simulink subsystem "SimscapePlantModels"  (R2023b)
settings: Solver=VariableStepAuto  StartTime=0.0  StopTime=10.0  RelTol=1e-3
undefined symbols (not defined in the file or in its folder): AxlFL, AxlFR, AxlRL, AxlRR, PlntTrnsfrCaseAxlSpdLock, PlntTrnsfrCaseTrqSplitRatio
libraries: fl_lib x13, nesl_utility_internal x9, sdl_lib x3, simulink x2, nesl_utility x2
(part 1 of 2)
settings Model: ModifiedByFormat=The MathWorks, Inc.  Creator=The MathWorks, Inc.  LastModifiedBy=The MathWorks, Inc.
settings SolverCC: MaxZcPerStep=1
settings OptimizationCC: ReuseModelBlockBuffer=off
settings DebuggingCC: UnconnectedInputMsg=warning  UnconnectedOutputMsg=warning  UnconnectedLineMsg=warning  SubsystemReferenceDiagnosticForUnitTest=warning
settings ModelReferenceCC: EnableRefExpFcnMdlSchedulingChecks=on
settings RTWCC: DLArmComputeVersion=19.05

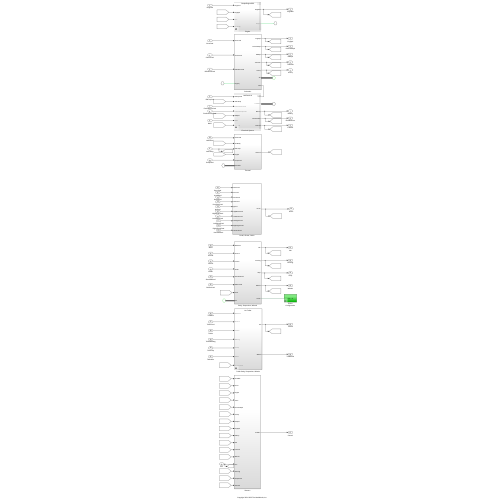
[thumbnail: Simulink's stored preview of the top-level diagram]
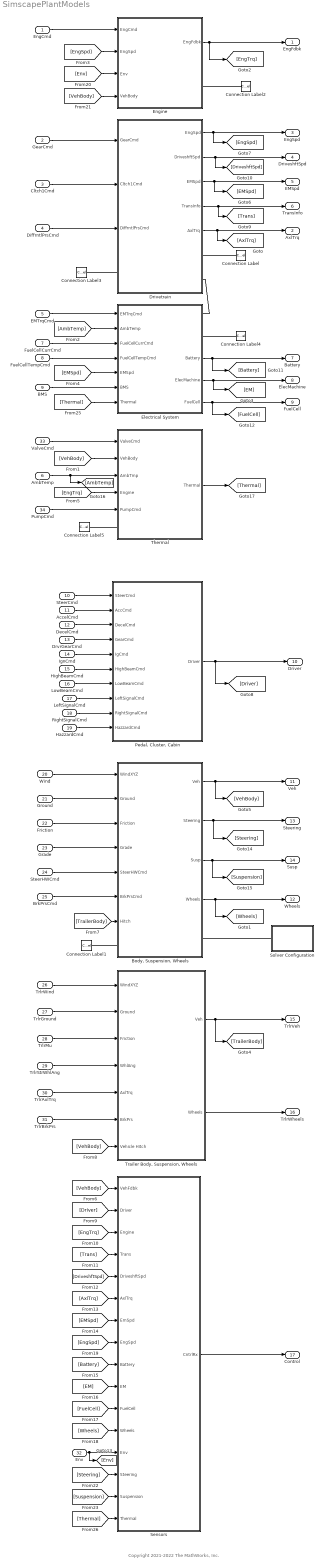
== system SimscapePlantModels ==
  note: Copyright 2021-2022 The MathWorks, Inc.
  EngCmd : Inport
  GearCmd : Inport  Port=2
  Cltch1Cmd : Inport  Port=3
  DiffrntlPrsCmd : Inport  Port=4
  EMTrqCmd : Inport  Port=5
  AmbTemp : Inport  Port=6
  FuelCellCurrCmd : Inport  Port=7
  FuelCellTempCmd : Inport  Port=8
  BMS : Inport  Port=9
  SteerCmd : Inport  Port=10
  AccelCmd : Inport  Port=11
  DecelCmd : Inport  Port=12
  DrvrGearCmd : Inport  Port=13
  IgnCmd : Inport  Port=14
  HighBeamCmd : Inport  Port=15
  LowBeamCmd : Inport  Port=16
  LeftSignalCmd : Inport  Port=17
  RightSignalCmd : Inport  Port=18
  HazzardCmd : Inport  Port=19
  Wind : Inport  Port=20
  Ground : Inport  Port=21
  Friction : Inport  Port=22
  Grade : Inport  Port=23
  SteerHWCmd : Inport  Port=24
  BrkPrsCmd : Inport  Port=25
  TrlrWind : Inport  Port=26
  TrlrGround : Inport  Port=27
  TrlrMu : Inport  Port=28
  TrlrStrWhlAng : Inport  Port=29
  TrlrAxlTrq : Inport  Port=30
  TrlrBrkPrs : Inport  Port=31
  Env : Inport  Port=32
  ValveCmd : Inport  Port=33
  PumpCmd : Inport  Port=34
  "Body, Suspension, Wheels" : Subsystem  VariantControl=Longitudinal Vehicle Dynamics
  Connection Label : ConnectionLabel  Label=Axl
  Connection Label1 : ConnectionLabel  Label=Axl
  Connection Label2 : ConnectionLabel  Label=EngTrq
  Connection Label3 : ConnectionLabel  Label=EngTrq
  Connection Label4 : ConnectionLabel  Label=ThrmElec
  Connection Label5 : ConnectionLabel  Label=ThrmElec
  Drivetrain : Subsystem
  Electrical System : Subsystem  Variant=on  VariantChoicesSpecifier={'ElectricalSystemSSC', 'NoElectrical'}  VariantControlMode=label  VariantControl=Choice  LabelModeActiveChoice=NoElectrical
      settings: PortSchema="{\"entries\":[{\"content\":{\"sides\":[{\"content\":{\"connectorIds\":[\"In1\",\"In2\",\"In3\",\"In4\",\"In5\",\"In6\",\"In7\"]},\"type\":\"ConnectorPlacement.EquallySpacedRectSide\",\"uuid\":\"168fda7d-02fd-4045-80e4-d70d0b749a9c\"},{\"content\":{\"connectorIds\":[\"RConn1\",\"RConn2\",\"Out1\",\"Out2\",\"Out3\"],\"side\":\"RIGHT\"},\"type\":\"ConnectorPlacement.EquallySpacedRectSide\",\"uuid\":\"a7e9bf4a-b9ce-46d6-8afc-0075c6e03a0c\"},{\"content\":{\"side\":\"TOP\"},\"type\":\"ConnectorPlacement.EquallySpacedRectSide\",\"uuid\":\"81c60468-d7ed-4851-a727-3a9a5b008640\"}]},\"type\":\"ConnectorPlacement.EquallySpacedConnector\",\"uuid\":\"8c7c8f28-264e-479c-b2d0-01b49dca4966\"}],\"packageUris\":[\"http://schema.mathworks.com/mf0/Connector/R2020b\"],\"version\":\"1.0\"}"
  Engine : Subsystem  Variant=on  VariantChoicesSpecifier={'FMUEngineSSC', 'NoEngine', 'SimpleEngineSSC'}  VariantControlMode=label  LabelModeActiveChoice=SimpleEngineSSC
  "Pedal, Cluster, Cabin" : Subsystem
  Sensors : Subsystem
  Solver Configuration : Subsystem  Variant=on  VariantControlMode=label  VariantControl=Choice  LabelModeActiveChoice=Solver Configuration
  Thermal : Subsystem
  "Trailer Body, Suspension, Wheels" : Subsystem  Variant=on  VariantControlMode=label  LabelModeActiveChoice=No Trailer
  EngFdbk : Outport
  AxlTrq : Outport  Port=2
  EngSpd : Outport  Port=3
  DriveshftSpd : Outport  Port=4
  EMSpd : Outport  Port=5
  TransInfo : Outport  Port=6
  Battery : Outport  Port=7
  ElecMachine : Outport  Port=8
  FuelCell : Outport  Port=9
  Driver : Outport  Port=10
  Veh : Outport  Port=11
  Wheels : Outport  Port=12
  Steering : Outport  Port=13
  Susp : Outport  Port=14
  TrlrVeh : Outport  Port=15
  TrlrWheels : Outport  Port=16
  Control : Outport  Port=17
  wires:
  Drivetrain/4(TransInfo) -> [Trans], TransInfo/1
  EngCmd/1 -> Engine/1(EngCmd)
  Electrical System/3(FuelCell) -> FuelCell/1, [FuelCell]
  Electrical System/1(Battery) -> Battery/1, [Battery]
  TrlrGround/1 -> "Trailer Body, Suspension, Wheels"/2(Ground)
  Wind/1 -> "Body, Suspension, Wheels"/1(WindXYZ)
  TrlrAxlTrq/1 -> "Trailer Body, Suspension, Wheels"/5(AxlTrq)
  EMTrqCmd/1 -> Electrical System/1(EMTrqCmd)
  DiffrntlPrsCmd/1 -> Drivetrain/3(DiffrntlPrsCmd)
  TrlrMu/1 -> "Trailer Body, Suspension, Wheels"/3(Friction)
  Friction/1 -> "Body, Suspension, Wheels"/3(Friction)
  SteerHWCmd/1 -> "Body, Suspension, Wheels"/5(SteerHWCmd)
  [EMSpd] -> Electrical System/5(EMSpd)
  Ground/1 -> "Body, Suspension, Wheels"/2(Ground)
  SteerCmd/1 -> "Pedal, Cluster, Cabin"/1(SteerCmd)
  TrlrBrkPrs/1 -> "Trailer Body, Suspension, Wheels"/6(BrkPrs)
  Drivetrain/2(DriveshftSpd) -> [DriveshftSpd], DriveshftSpd/1
  "Body, Suspension, Wheels"/1(Veh) -> [VehBody], Veh/1
  Engine/1(EngFdbk) -> [EngTrq], EngFdbk/1
  BrkPrsCmd/1 -> "Body, Suspension, Wheels"/6(BrkPrsCmd)
  Cltch1Cmd/1 -> Drivetrain/2(Cltch1Cmd)
  TrlrWind/1 -> "Trailer Body, Suspension, Wheels"/1(WindXYZ)
  TrlrStrWhlAng/1 -> "Trailer Body, Suspension, Wheels"/4(WhlAng)
  [VehBody] -> "Trailer Body, Suspension, Wheels"/7(Vehicle Hitch)
  "Trailer Body, Suspension, Wheels"/2(Wheels) -> TrlrWheels/1
  Electrical System/2(ElecMachine) -> ElecMachine/1, [EM]
  [TrailerBody] -> "Body, Suspension, Wheels"/7(Hitch)
  DecelCmd/1 -> "Pedal, Cluster, Cabin"/3(DecelCmd)
  DrvrGearCmd/1 -> "Pedal, Cluster, Cabin"/4(GearCmd)
  Drivetrain/3(EMSpd) -> [EMSpd], EMSpd/1
  IgnCmd/1 -> "Pedal, Cluster, Cabin"/5(IgCmd)
  FuelCellTempCmd/1 -> Electrical System/4(FuelCellTempCmd)
  GearCmd/1 -> Drivetrain/1(GearCmd)
  "Body, Suspension, Wheels"/4(Wheels) -> [Wheels], Wheels/1
  "Trailer Body, Suspension, Wheels"/1(Veh) -> TrlrVeh/1, [TrailerBody]
  FuelCellCurrCmd/1 -> Electrical System/3(FuelCellCurrCmd)
  AccelCmd/1 -> "Pedal, Cluster, Cabin"/2(AccCmd)
  Drivetrain/1(EngSpd) -> EngSpd/1, [EngSpd]
  [VehBody] -> Sensors/1(VehFdbk)
  "Pedal, Cluster, Cabin"/1(Driver) -> Driver/1, [Driver]
  [Driver] -> Sensors/2(Driver)
  [EngTrq] -> Sensors/3(Engine)
  [Trans] -> Sensors/4(Trans)
  [DriveshftSpd] -> Sensors/5(DriveshftSpd)
  [AxlTrq] -> Sensors/6(AxlTrq)
  [EMSpd] -> Sensors/7(EmSpd)
  [Battery] -> Sensors/9(Battery)
  [EM] -> Sensors/10(EM)
  [FuelCell] -> Sensors/11(FuelCell)
  [Wheels] -> Sensors/12(Wheels)
  Sensors/1(CntrlRx) -> Control/1
  Env/1 -> [Env], Sensors/13(Env)
  [EngSpd] -> Sensors/8(EngSpd)
  [Env] -> Engine/3(Env)
  [VehBody] -> Engine/4(VehBody)
  [EngSpd] -> Engine/2(EngSpd)
  "Body, Suspension, Wheels"/3(Susp) -> [Suspension], Susp/1
  Grade/1 -> "Body, Suspension, Wheels"/4(Grade)
  Drivetrain/5(AxlTrq) -> [AxlTrq], AxlTrq/1
  BMS/1 -> Electrical System/6(BMS)
  [Steering] -> Sensors/14(Steering)
  [Suspension] -> Sensors/15(Suspension)
  "Body, Suspension, Wheels"/2(Steering) -> [Steering], Steering/1
  Thermal/1(Thermal) -> [Thermal]
  [VehBody] -> Thermal/2(VehBody)
  ValveCmd/1 -> Thermal/1(ValveCmd)
  [EngTrq] -> Thermal/4(Engine)
  AmbTemp/1 -> [AmbTemp], Thermal/3(AmbTmp)
  [AmbTemp] -> Electrical System/2(AmbTemp)
  [Thermal] -> Electrical System/7(Thermal)
  [Thermal] -> Sensors/16(Thermal)
  PumpCmd/1 -> Thermal/5(PumpCmd)
  RightSignalCmd/1 -> "Pedal, Cluster, Cabin"/9(RightSignalCmd)
  LowBeamCmd/1 -> "Pedal, Cluster, Cabin"/7(LowBeamCmd)
  HighBeamCmd/1 -> "Pedal, Cluster, Cabin"/6(HighBeamCmd)
  HazzardCmd/1 -> "Pedal, Cluster, Cabin"/10(HazzardCmd)
  LeftSignalCmd/1 -> "Pedal, Cluster, Cabin"/8(LeftSignalCmd)
  connections:
  Connection Label/LConn1 -- Drivetrain/RConn1
  "Body, Suspension, Wheels"/LConn1 -- Connection Label1/LConn1
  Electrical System/RConn1 -- Drivetrain/RConn2
  Drivetrain/LConn1 -- Connection Label3/LConn1
  Connection Label2/LConn1 -- Engine/RConn1
  Solver Configuration/RConn1 -- "Body, Suspension, Wheels"/RConn1
  Thermal/LConn1 -- Connection Label5/LConn1
  Connection Label4/LConn1 -- Electrical System/RConn2

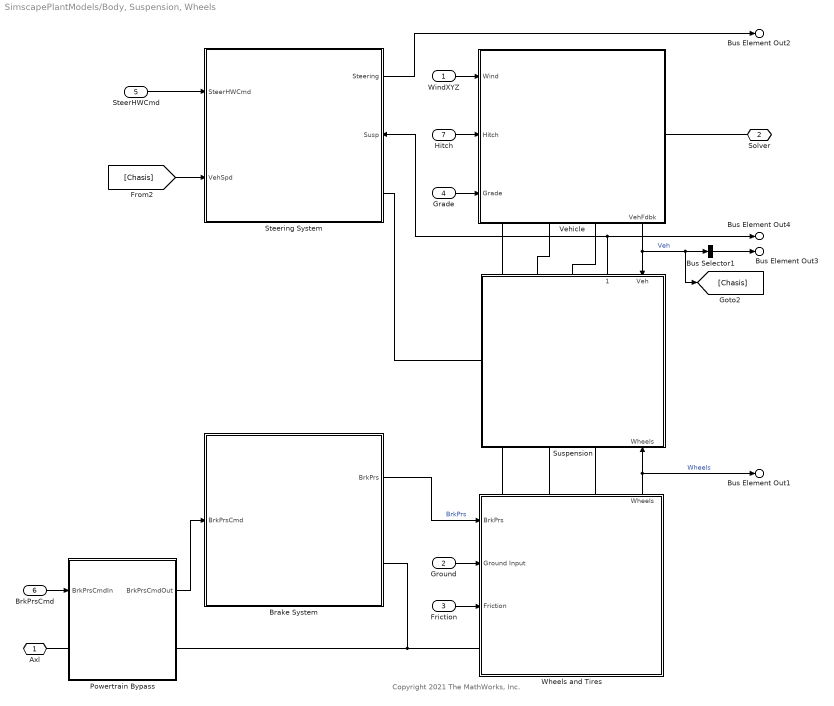
== system SimscapePlantModels/Body, Suspension, Wheels ==
  note: Copyright 2021 The MathWorks, Inc.
  WindXYZ : Inport  Unit=m/s  PortDimensions=3
  Ground : Inport  Port=2  Unit=m  PortDimensions=4
  Friction : Inport  Port=3  Unit=1  PortDimensions=4
  Grade : Inport  Port=4  Unit=deg  PortDimensions=1
  SteerHWCmd : Inport  Port=5  Unit=rad
  BrkPrsCmd : Inport  Port=6  PortDimensions=4
  Hitch : Inport  Port=7
  Brake System : Subsystem  Variant=on  VariantControlMode=label  VariantControl=Choice  LabelModeActiveChoice=Braking Hydraulics and Disc Brakes
      mask Display: image('Caliper.png',[.125,.125,.75,.75])
  Bus Selector1 : BusSelector  OutputSignals=InertFrm,BdyFrm  OutputAsBus=on
  Powertrain Bypass : Subsystem  Variant=on  VariantControlMode=label  VariantControl=Choice  LabelModeActiveChoice=Pass Through
  Steering System : Subsystem  Variant=on  VariantChoicesSpecifier={'NoSteering', 'SteeringSystemSSC'}  VariantControlMode=label  VariantControl=0  LabelModeActiveChoice=NoSteering
      settings: PortSchema="{\"entries\":[{\"content\":{\"sides\":[{\"content\":{\"connectorIds\":[\"In1\",\"In2\"]},\"type\":\"ConnectorPlacement.EquallySpacedRectSide\",\"uuid\":\"f4eae9a1-ee72-4894-9c3f-d81ee40fba89\"},{\"content\":{\"connectorIds\":[\"Out1\",\"In3\",\"RConn1\"],\"side\":\"RIGHT\"},\"type\":\"ConnectorPlacement.EquallySpacedRectSide\",\"uuid\":\"c62a78d9-dc5d-4f96-a554-c82d7fa22a9e\"},{\"content\":{\"side\":\"TOP\"},\"type\":\"ConnectorPlacement.EquallySpacedRectSide\",\"uuid\":\"38f3851a-1d1e-4a2b-8c09-8e5c8dcc7723\"}]},\"type\":\"ConnectorPlacement.EquallySpacedConnector\",\"uuid\":\"9f269846-92fa-4948-bc2b-71154f41fdde\"}],\"packageUris\":[\"http://schema.mathworks.com/mf0/Connector/R2020b\"],\"version\":\"1.0\"}"
      mask Display:
      | switch get_param(gcb,'ActiveVariant')
      |     case 'Kinematic Steering'
      |         image('KinematicSteering.png');
      |     case 'Mapped Steering'
      |         image('MappedSteering.png');
      |     case 'Dynamic Steering'
      |         image('DynamicSteering.png');
      |     otherwise
      |         image('DynamicSteering.png');
      | end
  Suspension : Subsystem  Variant=on  VariantChoicesSpecifier={'MultibodySuspensionSSC', 'NoSuspensionSSC'}  VariantControlMode=label  VariantControl=Choice  LabelModeActiveChoice=NoSuspensionSSC
      settings: PortSchema="{\"entries\":[{\"content\":{\"sides\":[{\"content\":{\"connectorIds\":[\"LConn1\"]},\"type\":\"ConnectorPlacement.EquallySpacedRectSide\",\"uuid\":\"0a9265e3-f55e-4b74-9b74-681dc9522591\"},{\"content\":{\"side\":\"RIGHT\"},\"type\":\"ConnectorPlacement.EquallySpacedRectSide\",\"uuid\":\"92df639a-7bc2-4e90-97ea-0cb216e2f16a\"},{\"content\":{\"connectorIds\":[\"LConn2\",\"LConn3\",\"LConn4\",\"Out1\",\"In1\"],\"side\":\"TOP\"},\"type\":\"ConnectorPlacement.EquallySpacedRectSide\",\"uuid\":\"2064b6cb-c7a8-4cfb-82de-a07750d990cb\"},{\"content\":{\"connectorIds\":[\"RConn1\",\"RConn2\",\"RConn3\",\"In2\"],\"side\":\"BOTTOM\"},\"type\":\"ConnectorPlacement.EquallySpacedRectSide\",\"uuid\":\"169bd4e6-c3fe-4e36-acea-c25875014463\"}]},\"type\":\"ConnectorPlacement.EquallySpacedConnector\",\"uuid\":\"e0b50182-0637-4594-80e7-4ddd0df85797\"}],\"packageUris\":[\"http://schema.mathworks.com/mf0/Connector/R2020b\"],\"version\":\"1.0\"}"
      mask Display:
      | switch get_param(gcb,'ActiveVariant')
      |     case 'Kinematics and Compliance Independent Suspension'
      |         image('KandCSuspension.png');
      |     case 'Kinematics and Compliance Twist Beam Suspension'
      |         image('KandCSuspensionTwistBeam.png');
      |     case 'MacPherson Front Suspension Solid Axle Rear Suspension'
      |         image([imread('suspmacp.png');imread('suspsacoil.png')]);
      |     otherwise
      |         image([imread('suspmacp.png');imread('suspsacoil.png')]);
      | end
  Vehicle : Subsystem  Variant=on  VariantChoicesSpecifier={'VehicleBody1DOFLongitudinalSSC', 'VehicleBody3DOFLongitudinalSSC', 'VehicleBody6DOFSSC'}  VariantControlMode=label  VariantControl=Choice  LabelModeActiveChoice=VehicleBody3DOFLongitudinalSSC
      settings: PortSchema="{\"entries\":[{\"content\":{\"sides\":[{\"content\":{\"connectorIds\":[\"In1\",\"In2\",\"In3\"]},\"type\":\"ConnectorPlacement.EquallySpacedRectSide\",\"uuid\":\"0a9265e3-f55e-4b74-9b74-681dc9522591\"},{\"content\":{\"connectorIds\":[\"RConn1\"],\"side\":\"RIGHT\"},\"type\":\"ConnectorPlacement.EquallySpacedRectSide\",\"uuid\":\"92df639a-7bc2-4e90-97ea-0cb216e2f16a\"},{\"content\":{\"connectorIds\":[],\"side\":\"TOP\"},\"type\":\"ConnectorPlacement.EquallySpacedRectSide\",\"uuid\":\"2064b6cb-c7a8-4cfb-82de-a07750d990cb\"},{\"content\":{\"connectorIds\":[\"RConn2\",\"RConn3\",\"RConn4\",\"Out1\"],\"side\":\"BOTTOM\"},\"type\":\"ConnectorPlacement.EquallySpacedRectSide\",\"uuid\":\"2b34afca-0a88-43db-924f-6476183b84bd\"}]},\"type\":\"ConnectorPlacement.EquallySpacedConnector\",\"uuid\":\"e0b50182-0637-4594-80e7-4ddd0df85797\"}],\"packageUris\":[\"http://schema.mathworks.com/mf0/Connector/R2020b\"],\"version\":\"1.0\"}"
      mask Display: image('6dofcar.png');
  Wheels and Tires : Subsystem  Variant=on  VariantChoicesSpecifier={'MFTiresLongitudinalSSC', 'MFTiresMultibodySSC'}  VariantControlMode=label  VariantControl=Choice  LabelModeActiveChoice=MFTiresLongitudinalSSC
      settings: PortSchema="{\"entries\":[{\"content\":{\"sides\":[{\"content\":{\"connectorIds\":[\"In1\",\"In2\",\"In3\",\"LConn1\"]},\"type\":\"ConnectorPlacement.EquallySpacedRectSide\",\"uuid\":\"fdb4d4cd-d0c0-42d9-b073-775af31e96a1\"},{\"content\":{\"connectorIds\":[],\"side\":\"RIGHT\"},\"type\":\"ConnectorPlacement.EquallySpacedRectSide\",\"uuid\":\"04106ddf-9917-4cd4-b177-ae763d642686\"},{\"content\":{\"connectorIds\":[\"LConn2\",\"LConn3\",\"LConn4\",\"Out1\"],\"side\":\"TOP\"},\"type\":\"ConnectorPlacement.EquallySpacedRectSide\",\"uuid\":\"568bf95c-0e25-4c45-a134-c198357b75be\"}]},\"type\":\"ConnectorPlacement.EquallySpacedConnector\",\"uuid\":\"4f44df5e-0d14-43ea-934e-2abe86546e95\"}],\"packageUris\":[\"http://schema.mathworks.com/mf0/Connector/R2020b\"],\"version\":\"1.0\"}"
      mask Display: image('wheel3dof.png')
  Axl : PMIOPort  Side=Left
  Solver : PMIOPort  Port=2  Side=Right
  Bus Element Out3 : Outport  PortName=Veh
  Bus Element Out2 : Outport  Port=2  PortName=Steering
  Bus Element Out4 : Outport  Port=3  PortName=Susp
  Bus Element Out1 : Outport  Port=4  PortName=Wheels
  wires:
  SteerHWCmd/1 -> Steering System/1(SteerHWCmd)
  Bus Selector1/1 -> Bus Element Out3/1
  WindXYZ/1 -> Vehicle/1(Wind)
  Brake System/1(BrkPrs) -> Wheels and Tires/1(BrkPrs)  "BrkPrs"
  Suspension/1(SuspChassis) -> Bus Element Out4/1, Steering System/3(Susp)
  Powertrain Bypass/1(BrkPrsCmdOut) -> Brake System/1(BrkPrsCmd)
  Wheels and Tires/1(Wheels) -> Bus Element Out1/1, Suspension/2(Wheels)  "Wheels"
  Grade/1 -> Vehicle/3(Grade)
  Hitch/1 -> Vehicle/2(Hitch)
  Friction/1 -> Wheels and Tires/3(Friction)
  Steering System/1(Steering) -> Bus Element Out2/1
  [Chasis] -> Steering System/2(VehSpd)
  Ground/1 -> Wheels and Tires/2(Ground Input)
  Vehicle/1(VehFdbk) -> [Chasis], Bus Selector1/1, Suspension/1(Veh)  "Veh"
  BrkPrsCmd/1 -> Powertrain Bypass/1(BrkPrsCmdIn)
  connections:
  Brake System/RConn1 -- Powertrain Bypass/RConn1 -- Wheels and Tires/LConn1
  Vehicle/RConn2 -- Suspension/LConn2
  Vehicle/RConn3 -- Suspension/LConn3
  Vehicle/RConn4 -- Suspension/LConn4
  Wheels and Tires/LConn2 -- Suspension/RConn1
  Wheels and Tires/LConn3 -- Suspension/RConn2
  Wheels and Tires/LConn4 -- Suspension/RConn3
  Vehicle/RConn1 -- Solver/RConn1
  Axl/RConn1 -- Powertrain Bypass/LConn1
  Steering System/RConn1 -- Suspension/LConn1

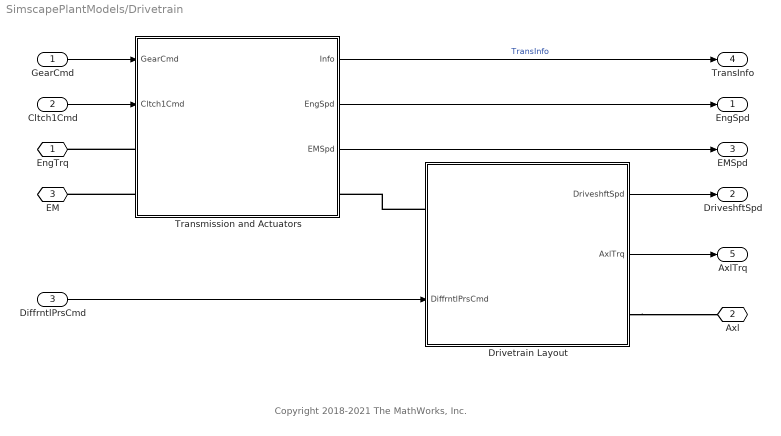
== system SimscapePlantModels/Drivetrain ==
  note: Copyright 2018-2021 The MathWorks, Inc.
  GearCmd : Inport
  Cltch1Cmd : Inport  Port=2
  DiffrntlPrsCmd : Inport  Port=3
  Drivetrain Layout : Subsystem  VariantControl=New
      settings: PortSchema="{\"entries\":[{\"content\":{\"sides\":[{\"content\":{\"connectorIds\":[\"LConn1\",\"In1\"]},\"type\":\"ConnectorPlacement.EquallySpacedRectSide\",\"uuid\":\"aca18566-8f68-4dbe-a1ea-7891e9b0f8a0\"},{\"content\":{\"connectorIds\":[\"Out1\",\"Out2\",\"RConn1\"],\"side\":\"RIGHT\"},\"type\":\"ConnectorPlacement.EquallySpacedRectSide\",\"uuid\":\"80817b32-8ae2-43ef-bc82-fae1c7a772cb\"},{\"content\":{\"connectorIds\":[],\"side\":\"TOP\"},\"type\":\"ConnectorPlacement.EquallySpacedRectSide\",\"uuid\":\"fadb27fa-7a73-4d3f-b69d-888e371ed2d5\"}]},\"type\":\"ConnectorPlacement.EquallySpacedConnector\",\"uuid\":\"7287b0c1-67df-44d5-bf90-b5b5a04fa161\"}],\"packageUris\":[\"http://schema.mathworks.com/mf0/Connector/R2020b\"],\"version\":\"1.0\"}"
  Transmission and Actuators : Subsystem  Variant=on  VariantChoicesSpecifier={'BEV1EMSSC', 'BEV2EMSSC', 'BEV3EMSSC', 'BEV4EMSSC', 'ConventionalVehicleSSC', 'HEVIPSSSC', 'HEVMMSSC', 'HEVP0SSC', 'HEVP1SSC', 'HEVP2SSC', 'HEVP3SSC', 'HEVP4SSC'}  VariantControlMode=label  LabelModeActiveChoice=ConventionalVehicleSSC
  EngTrq : PMIOPort  Side=Left
  Axl : PMIOPort  Port=2  Side=Right
  EM : PMIOPort  Port=3  Side=Right
  EngSpd : Outport  Unit=rad/s  VectorParamsAs1DForOutWhenUnconnected=off
  DriveshftSpd : Outport  Port=2  VectorParamsAs1DForOutWhenUnconnected=off
  EMSpd : Outport  Port=3  Unit=rad/s  VectorParamsAs1DForOutWhenUnconnected=off
  TransInfo : Outport  Port=4  VectorParamsAs1DForOutWhenUnconnected=off
  AxlTrq : Outport  Port=5  VectorParamsAs1DForOutWhenUnconnected=off
  wires:
  Transmission and Actuators/1(Info) -> TransInfo/1  "TransInfo"
  DiffrntlPrsCmd/1 -> Drivetrain Layout/1(DiffrntlPrsCmd)
  Cltch1Cmd/1 -> Transmission and Actuators/2(Cltch1Cmd)
  Drivetrain Layout/1(DriveshftSpd) -> DriveshftSpd/1
  GearCmd/1 -> Transmission and Actuators/1(GearCmd)
  Transmission and Actuators/2(EngSpd) -> EngSpd/1
  Transmission and Actuators/3(EMSpd) -> EMSpd/1
  Drivetrain Layout/2(AxlTrq) -> AxlTrq/1
  connections:
  Transmission and Actuators/LConn2 -- EM/RConn1
  Drivetrain Layout/RConn1 -- Axl/RConn1
  Drivetrain Layout/LConn1 -- Transmission and Actuators/RConn1
  Transmission and Actuators/LConn1 -- EngTrq/RConn1

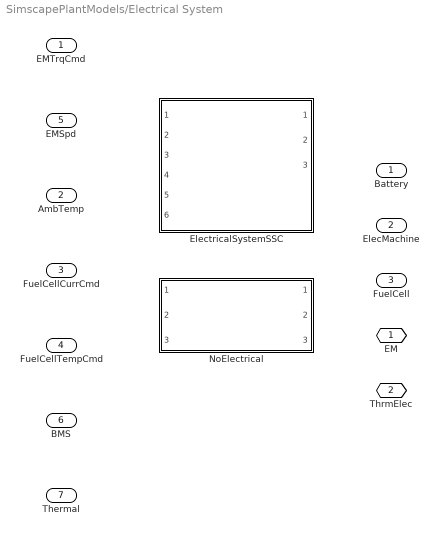
== system SimscapePlantModels/Electrical System ==
  EMTrqCmd : Inport
  AmbTemp : Inport  Port=2
  FuelCellCurrCmd : Inport  Port=3
  FuelCellTempCmd : Inport  Port=4
  EMSpd : Inport  Port=5
  BMS : Inport  Port=6
  Thermal : Inport  Port=7
  ElectricalSystemSSC : Subsystem  VariantControl=ElectricalSystemSSC  ReferencedSubsystem=ElectricalSystemSSC
  NoElectrical : Subsystem  VariantControl=NoElectrical  ReferencedSubsystem=NoElectrical
  EM : PMIOPort  Side=Right
  ThrmElec : PMIOPort  Port=2  Side=Right
  Battery : Outport
  ElecMachine : Outport  Port=2
  FuelCell : Outport  Port=3

== system SimscapePlantModels/Engine ==
  EngCmd : Inport
  EngSpd : Inport  Port=2
  Env : Inport  Port=3
  VehBody : Inport  Port=4
  FMUEngineSSC : Subsystem  VariantControl=FMUEngineSSC  ReferencedSubsystem=FMUEngineSSC
  NoEngine : Subsystem  VariantControl=NoEngine  ReferencedSubsystem=NoEngine
  SimpleEngineSSC : Subsystem  VariantControl=SimpleEngineSSC  ReferencedSubsystem=SimpleEngineSSC
  EngTrq : PMIOPort  Side=Right
  EngFdbk : Outport  VectorParamsAs1DForOutWhenUnconnected=off

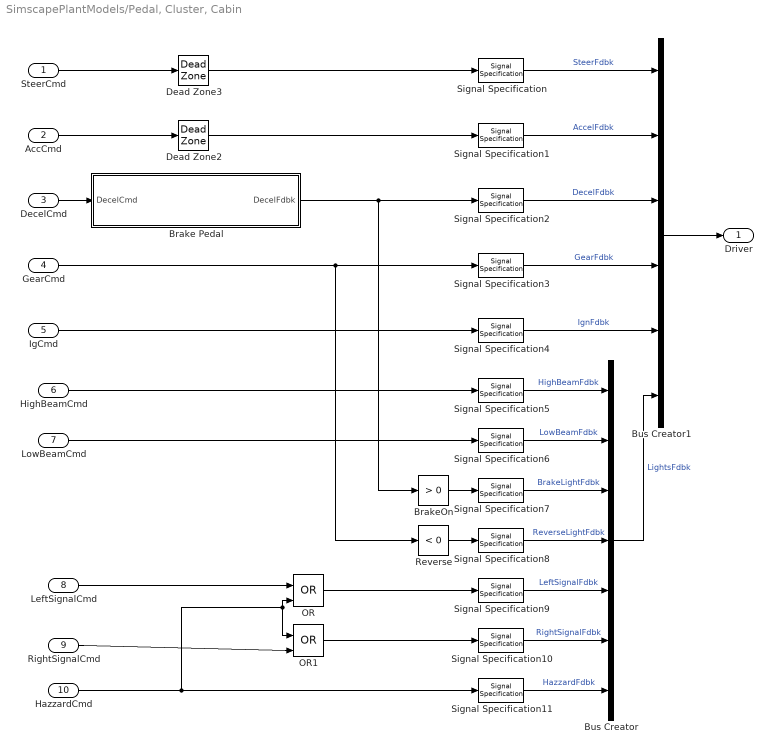
== system SimscapePlantModels/Pedal, Cluster, Cabin ==
  SteerCmd : Inport
  AccCmd : Inport  Port=2
  DecelCmd : Inport  Port=3
  GearCmd : Inport  Port=4
  IgCmd : Inport  Port=5
  HighBeamCmd : Inport  Port=6
  LowBeamCmd : Inport  Port=7
  LeftSignalCmd : Inport  Port=8
  RightSignalCmd : Inport  Port=9
  HazzardCmd : Inport  Port=10
  Brake Pedal : Subsystem
  BrakeOn : simulink/Logic and Bit Operations/Compare To Constant  relop=>  const=0  OutDataTypeStr=boolean  ZeroCross=off
  Bus Creator : BusCreator  Inputs=7
  Bus Creator1 : BusCreator  Inputs=6
  Dead Zone2 : DeadZone  LowerValue=0  UpperValue=.01  ZeroCross=off
  Dead Zone3 : DeadZone  LowerValue=-.01  UpperValue=.01  ZeroCross=off
  OR : Logic  Operator=OR  IconShape=distinctive  AllPortsSameDT=off  OutDataTypeStr=boolean
  OR1 : Logic  Operator=OR  IconShape=distinctive  AllPortsSameDT=off  OutDataTypeStr=boolean
  Reverse : simulink/Logic and Bit Operations/Compare To Constant  relop=<  const=0  OutDataTypeStr=boolean  ZeroCross=off
  Signal Specification : SignalSpecification  Unit=rad
  Signal Specification{1..11} (11 alike) : SignalSpecification  Unit=1
  Driver : Outport
  wires:
  Signal Specification9/1 -> Bus Creator/5  "LeftSignalFdbk"
  Signal Specification11/1 -> Bus Creator/7  "HazzardFdbk"
  Signal Specification10/1 -> Bus Creator/6  "RightSignalFdbk"
  Signal Specification8/1 -> Bus Creator/4  "ReverseLightFdbk"
  Signal Specification7/1 -> Bus Creator/3  "BrakeLightFdbk"
  Signal Specification6/1 -> Bus Creator/2  "LowBeamFdbk"
  Signal Specification5/1 -> Bus Creator/1  "HighBeamFdbk"
  Bus Creator/1 -> Bus Creator1/6  "LightsFdbk"
  RightSignalCmd/1 -> OR1/2
  LowBeamCmd/1 -> Signal Specification6/1
  HazzardCmd/1 -> OR1/1, OR/2, Signal Specification11/1
  LeftSignalCmd/1 -> OR/1
  Reverse/1 -> Signal Specification8/1
  OR/1 -> Signal Specification9/1
  OR1/1 -> Signal Specification10/1
  BrakeOn/1 -> Signal Specification7/1
  HighBeamCmd/1 -> Signal Specification5/1
  Dead Zone3/1 -> Signal Specification/1
  Signal Specification1/1 -> Bus Creator1/2  "AccelFdbk"
  Signal Specification4/1 -> Bus Creator1/5  "IgnFdbk"
  Brake Pedal/1(DecelFdbk) -> Signal Specification2/1, BrakeOn/1
  Signal Specification/1 -> Bus Creator1/1  "SteerFdbk"
  Signal Specification2/1 -> Bus Creator1/3  "DecelFdbk"
  GearCmd/1 -> Signal Specification3/1, Reverse/1
  Bus Creator1/1 -> Driver/1
  IgCmd/1 -> Signal Specification4/1
  Signal Specification3/1 -> Bus Creator1/4  "GearFdbk"
  Dead Zone2/1 -> Signal Specification1/1
  SteerCmd/1 -> Dead Zone3/1
  AccCmd/1 -> Dead Zone2/1
  DecelCmd/1 -> Brake Pedal/1(DecelCmd)

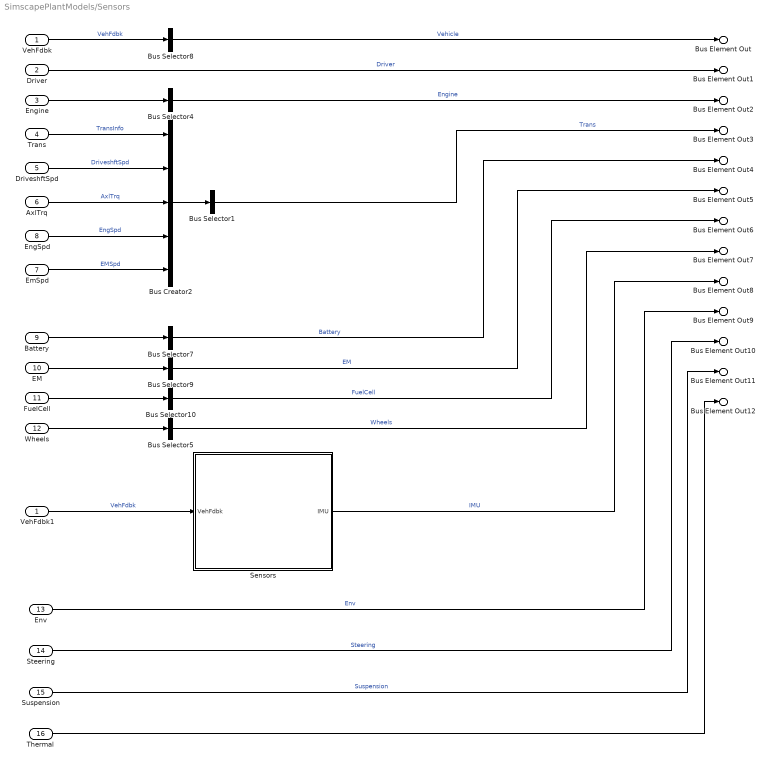
== system SimscapePlantModels/Sensors ==
  VehFdbk : Inport
  Driver : Inport  Port=2
  Engine : Inport  Port=3
  Trans : Inport  Port=4
  DriveshftSpd : Inport  Port=5
  AxlTrq : Inport  Port=6
  EmSpd : Inport  Port=7
  EngSpd : Inport  Port=8
  Battery : Inport  Port=9
  EM : Inport  Port=10
  FuelCell : Inport  Port=11
  Wheels : Inport  Port=12
  Env : Inport  Port=13
  Steering : Inport  Port=14
  Suspension : Inport  Port=15
  Thermal : Inport  Port=16
  Bus Creator2 : BusCreator  Inputs=5
  Bus Selector1 : BusSelector  OutputSignals=TransInfo.Cltch1State,TransInfo.Cltch2State,DriveshftSpd,AxlTrq,EngSpd,EMSpd,TransInfo.TransInfo.Trans.TransGear  OutputAsBus=on
  Bus Selector10 : BusSelector  OutputSignals=FuelCellVolt,FuelCellCurr,H2Flw  OutputAsBus=on
  Bus Selector4 : BusSelector  OutputSignals=EngTrq,Map,Mat,ThrPosPct,WgAreaPct,IntkCamPhase,ExhCamPhase,TurboRackPos,EgrVlvAreaPct,VarCompRatioPos,IntkVlvLift,VarIntkRunLen,Afr,IntkSwirlVlvPos,TurboSpd,Iat,Ect,EgrVlvDeltaPrs,EgrVlvInTemp  OutputAsBus=on
  Bus Selector5 : BusSelector  OutputSignals=Wheels.BrkPrs,Wheels.Kappa,Wheels.Alpha,Wheels.Omega  OutputAsBus=on
  Bus Selector7 : BusSelector  OutputSignals=BattSoc,BattVolt,BattCurr,BattPwr,BMSSensors  OutputAsBus=on
  Bus Selector8 : BusSelector  OutputSignals=BdyFrm.Cg.Vel.xdot,BdyFrm.Cg.Acc.ax,BdyFrm.Cg.Acc.xddot  OutputAsBus=on
  Bus Selector9 : BusSelector  OutputSignals=EMTrq,EMPwrElec  OutputAsBus=on
  Sensors : Subsystem  Variant=on  VariantChoicesSpecifier={'IMUSensor', 'NoIMUSensor'}  VariantControlMode=label  VariantControl=Choice  LabelModeActiveChoice=NoIMUSensor
  VehFdbk1 : InportShadow
  Bus Element Out : Outport  PortName=CntrlRx  Element=Vehicle
  Bus Element Out1 : Outport  PortName=CntrlRx  Element=Driver
  Bus Element Out2 : Outport  PortName=CntrlRx  Element=Engine
  Bus Element Out3 : Outport  PortName=CntrlRx  Element=Trans
  Bus Element Out4 : Outport  PortName=CntrlRx  Element=Battery
  Bus Element Out5 : Outport  PortName=CntrlRx  Element=EM
  Bus Element Out6 : Outport  PortName=CntrlRx  Element=FuelCell
  Bus Element Out7 : Outport  PortName=CntrlRx  Element=Wheels
  Bus Element Out8 : Outport  PortName=CntrlRx  Element=IMU
  Bus Element Out9 : Outport  PortName=CntrlRx  Element=Env
  Bus Element Out10 : Outport  PortName=CntrlRx  Element=Steering
  Bus Element Out11 : Outport  PortName=CntrlRx  Element=Suspension
  Bus Element Out12 : Outport  PortName=CntrlRx  Element=Thermal
  wires:
  Bus Selector1/1 -> Bus Element Out3/1  "Trans"
  Bus Creator2/1 -> Bus Selector1/1
  Trans/1 -> Bus Creator2/1  "TransInfo"
  EngSpd/1 -> Bus Creator2/4  "EngSpd"
  Env/1 -> Bus Element Out9/1  "Env"
  Driver/1 -> Bus Element Out1/1  "Driver"
  Sensors/1(IMU) -> Bus Element Out8/1  "IMU"
  VehFdbk1/1 -> Sensors/1(VehFdbk)  "VehFdbk"
  Wheels/1 -> Bus Selector5/1
  FuelCell/1 -> Bus Selector10/1
  EM/1 -> Bus Selector9/1
  Battery/1 -> Bus Selector7/1
  EmSpd/1 -> Bus Creator2/5  "EMSpd"
  AxlTrq/1 -> Bus Creator2/3  "AxlTrq"
  DriveshftSpd/1 -> Bus Creator2/2  "DriveshftSpd"
  Engine/1 -> Bus Selector4/1
  VehFdbk/1 -> Bus Selector8/1  "VehFdbk"
  Bus Selector4/1 -> Bus Element Out2/1  "Engine"
  Bus Selector10/1 -> Bus Element Out6/1  "FuelCell"
  Bus Selector9/1 -> Bus Element Out5/1  "EM"
  Bus Selector8/1 -> Bus Element Out/1  "Vehicle"
  Bus Selector7/1 -> Bus Element Out4/1  "Battery"
  Bus Selector5/1 -> Bus Element Out7/1  "Wheels"
  Steering/1 -> Bus Element Out10/1  "Steering"
  Suspension/1 -> Bus Element Out11/1  "Suspension"
  Thermal/1 -> Bus Element Out12/1

== system SimscapePlantModels/Solver Configuration ==
  Local Solver : nesl_utility/Solver Configuration  VariantControl=Local Solver  PhysicalDomain=network_engine_domain  SubClassName=solver  LeftPortType=input  RightPortType=generic  Tones=[]  Harmonics=[]  SimulateNoise=off  Profile=off  UseLocalSampling=off  EnableSwitchedLinearOptims=on  FrequencyDomain=off  UseCCode=off  RelTol=0.001  AbsTol=0.001  MinStep=1e-09  ToWorkspace=off  RevertToSquareIcSolve=off  NumHomotopyIterations=100  PhasorMode=off  PhasorModeNumHarmonics=1  ConsistencySolver=NEWTON_XTOL_AFTER_FTOL  IndexReductionMethod=DerivativeReplacement  DoDC=off  ResidualTolerance=1e-09  ConsistencyTolSource=LOCAL  ConsistencyAbsTol=0.001  ConsistencyRelTol=0.001  ConsistencyTolFactor=0.001  UseLocalSolver=on  LocalSolverChoice=NE_BACKWARD_EULER_ADVANCER  ResolveIndetEquations=on  FunctionEvalNumThread=1  LocalSolverSampleTime=0.1  DoFixedCost=off  MaxNonlinIter=3  MaxModeIter=2  ComputeImpulses=off  ImpulseIterations=2  LinearAlgebra=auto  LinearAlgebraNumThread=0  EquationFormulation=NE_TIME_EF  DelaysMemoryBudget=1024  AutomaticFiltering=on  FilteringTimeConstant=0.001  PartitionStorageMethod=AS_NEEDED  PartitionMemoryBudget=1024  PartitionMethod=ROBUST  MultibodyUseLocalSolver=off  MultibodyLocalSolverChoice=ODE1  MultibodyLocalSolverSampleTime=0.001
  Solver Configuration : nesl_utility/Solver Configuration  VariantControl=Solver Configuration  PhysicalDomain=network_engine_domain  SubClassName=solver  LeftPortType=input  RightPortType=generic  Tones=[]  Harmonics=[]  SimulateNoise=off  Profile=off  UseLocalSampling=off  EnableSwitchedLinearOptims=on  FrequencyDomain=off  UseCCode=off  RelTol=0.001  AbsTol=0.001  MinStep=1e-09  ToWorkspace=off  RevertToSquareIcSolve=off  NumHomotopyIterations=100  PhasorMode=off  PhasorModeNumHarmonics=1  ConsistencySolver=NEWTON_XTOL_AFTER_FTOL  IndexReductionMethod=DerivativeReplacement  DoDC=off  ResidualTolerance=1e-09  ConsistencyTolSource=LOCAL  ConsistencyAbsTol=0.001  ConsistencyRelTol=0.001  ConsistencyTolFactor=0.001  UseLocalSolver=off  LocalSolverChoice=NE_BACKWARD_EULER_ADVANCER  ResolveIndetEquations=on  FunctionEvalNumThread=1  LocalSolverSampleTime=0.001  DoFixedCost=off  MaxNonlinIter=3  MaxModeIter=2  ComputeImpulses=off  ImpulseIterations=2  LinearAlgebra=auto  LinearAlgebraNumThread=0  EquationFormulation=NE_TIME_EF  DelaysMemoryBudget=1024  AutomaticFiltering=on  FilteringTimeConstant=0.001  PartitionStorageMethod=AS_NEEDED  PartitionMemoryBudget=1024  PartitionMethod=ROBUST  MultibodyUseLocalSolver=off  MultibodyLocalSolverChoice=ODE1  MultibodyLocalSolverSampleTime=0.001
  a : PMIOPort  Side=Right

== system SimscapePlantModels/Thermal ==
  ValveCmd : Inport
  VehBody : Inport  Port=2
  AmbTmp : Inport  Port=3
  Engine : Inport  Port=4
  PumpCmd : Inport  Port=5
  Electrical Cooling : Subsystem  Variant=on  VariantControlMode=label  LabelModeActiveChoice=No Thermal Effect
  Terminator : Terminator
  ThrmElec : PMIOPort  Side=Left
  Thermal : Outport
  wires:
  AmbTmp/1 -> Electrical Cooling/3(AmbTmp)
  VehBody/1 -> Electrical Cooling/2(VehBody)
  ValveCmd/1 -> Electrical Cooling/1(ValveCmd)
  Electrical Cooling/1(Thermal) -> Thermal/1
  Engine/1 -> Terminator/1
  PumpCmd/1 -> Electrical Cooling/4(PumpCmd)
  connections:
  ThrmElec/RConn1 -- Electrical Cooling/LConn1

== system SimscapePlantModels/Trailer Body, Suspension, Wheels ==
  WindXYZ : Inport
  Ground : Inport  Port=2
  Friction : Inport  Port=3
  WhlAng : Inport  Port=4
  AxlTrq : Inport  Port=5
  BrkPrs : Inport  Port=6
  Vehicle Hitch : Inport  Port=7
  No Trailer : Subsystem  VariantControl=No Trailer
  One-Axle Trailer : Subsystem  VariantControl=One-Axle Trailer  ReferencedSubsystem=OneAxleTrailer
  Veh : Outport  VectorParamsAs1DForOutWhenUnconnected=off
  Wheels : Outport  Port=2  VectorParamsAs1DForOutWhenUnconnected=off

== system SimscapePlantModels/Body, Suspension, Wheels/Brake System ==
  BrkPrsCmd : Inport
  Braking Hydraulics and Disc Brakes : Subsystem  VariantControl=Braking Hydraulics and Disc Brakes  ReferencedSubsystem=BrakingHydraulicsDiscBrakesSSC
  Axl : PMIOPort  Side=Right
  BrkPrs : Outport

== system SimscapePlantModels/Body, Suspension, Wheels/Powertrain Bypass ==
  BrkPrsCmdIn : Inport
  External Signal Source : Subsystem  VariantControl=External Signal Source
  Pass Through : Subsystem  VariantControl=Pass Through
  AxlTrqIn : PMIOPort  Side=Left
  AxlTrqOut : PMIOPort  Port=2  Side=Right
  BrkPrsCmdOut : Outport

== system SimscapePlantModels/Body, Suspension, Wheels/Steering System ==
  SteerHWCmd : Inport
  VehSpd : Inport  Port=2
  Susp : Inport  Port=3
  NoSteering : Subsystem  VariantControl=NoSteering  ReferencedSubsystem=NoSteering
  SteeringSystemSSC : Subsystem  VariantControl=SteeringSystemSSC  ReferencedSubsystem=SteeringSystemSSC
  SteerSusp : PMIOPort  Side=Right
  Steering : Outport

== system SimscapePlantModels/Body, Suspension, Wheels/Suspension ==
  Veh : Inport
  Wheels : Inport  Port=2
  MultibodySuspensionSSC : Subsystem  VariantControl=MultibodySuspensionSSC  ReferencedSubsystem=MultibodySuspensionSSC
  NoSuspensionSSC : Subsystem  VariantControl=NoSuspensionSSC  ReferencedSubsystem=NoSuspensionSSC
  Steering : PMIOPort  Side=Left
  SuspVeh : PMIOPort  Port=2  Side=Left
  FrntAxlVeh : PMIOPort  Port=3  Side=Left
  RearAxlVeh : PMIOPort  Port=4  Side=Left
  SuspWhl : PMIOPort  Port=5  Side=Right
  FrntAxlWhl : PMIOPort  Port=6  Side=Right
  RearAxlWhl : PMIOPort  Port=7  Side=Right
  SuspChassis : Outport

== system SimscapePlantModels/Body, Suspension, Wheels/Vehicle ==
  Wind : Inport
  Hitch : Inport  Port=2
  Grade : Inport  Port=3
  VehicleBody1DOFLongitudinalSSC : Subsystem  VariantControl=VehicleBody1DOFLongitudinalSSC  ReferencedSubsystem=VehicleBody1DOFLongitudinalSSC
  VehicleBody3DOFLongitudinalSSC : Subsystem  VariantControl=VehicleBody3DOFLongitudinalSSC  ReferencedSubsystem=VehicleBody3DOFLongitudinalSSC
  VehicleBody6DOFSSC : Subsystem  VariantControl=VehicleBody6DOFSSC  ReferencedSubsystem=VehicleBody6DOFSSC
  Solver : PMIOPort  Side=Right
  SuspVeh : PMIOPort  Port=2  Side=Right
  FrntAxlVeh : PMIOPort  Port=3  Side=Right
  RearAxlVeh : PMIOPort  Port=4  Side=Right
  VehFdbk : Outport

== system SimscapePlantModels/Body, Suspension, Wheels/Wheels and Tires ==
  BrkPrs : Inport
  Ground Input : Inport  Port=2
  Friction : Inport  Port=3
  MFTiresLongitudinalSSC : Subsystem  VariantControl=MFTiresLongitudinalSSC  ReferencedSubsystem=MFTiresLongitudinalSSC
  MFTiresMultibodySSC : Subsystem  VariantControl=MFTiresMultibodySSC  ReferencedSubsystem=MFTiresMultibodySSC
  Axl : PMIOPort  Side=Left
  SuspWhl : PMIOPort  Port=2  Side=Left
  FrntAxlWhl : PMIOPort  Port=3  Side=Left
  RearAxlWhl : PMIOPort  Port=4  Side=Left
  Wheels : Outport

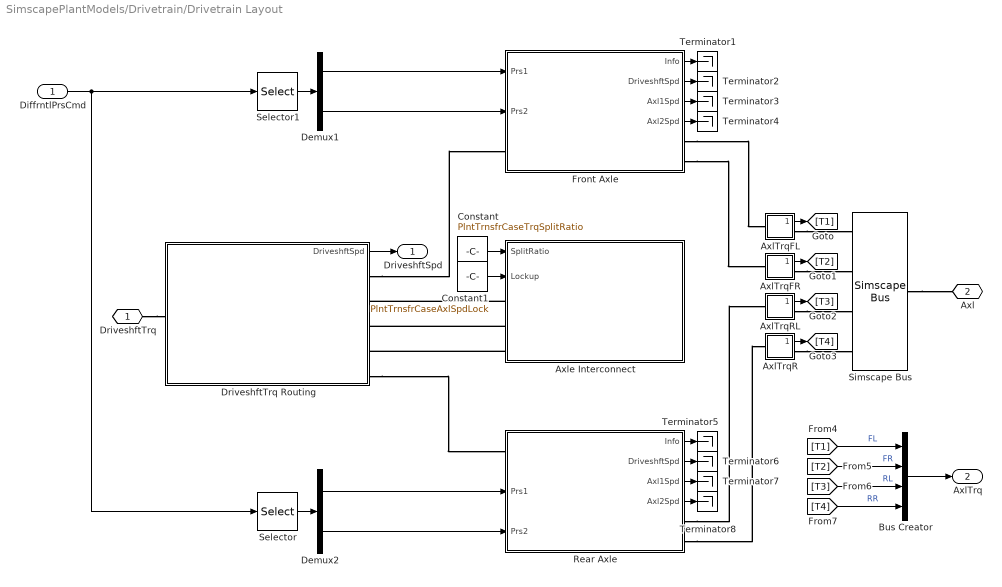
== system SimscapePlantModels/Drivetrain/Drivetrain Layout ==
  DiffrntlPrsCmd : Inport
  AxlTrqFL : Subsystem
  AxlTrqFR : Subsystem
  AxlTrqR : Subsystem
  AxlTrqRL : Subsystem
  Axle Interconnect : Subsystem  Variant=on  VariantChoicesSpecifier={'NoInterconnectSSC', 'TransferCaseSSC'}  VariantControlMode=label  VariantControl=Choice  LabelModeActiveChoice=NoInterconnectSSC
  Bus Creator : BusCreator  Inputs=4
  Constant : Constant  Value=PlntTrnsfrCaseTrqSplitRatio  SampleTime=-1
  Constant1 : Constant  Value=PlntTrnsfrCaseAxlSpdLock  SampleTime=-1
  Demux1 : Demux  Outputs=2
  Demux2 : Demux  Outputs=2
  DriveshftTrq Routing : Subsystem  Variant=on  VariantChoicesSpecifier={'FourActuatorAWDSSC', 'OneActuatorAWDSSC', 'OneActuatorFWDSSC', 'OneActuatorRWDSSC', 'ThreeActuatorAWD2EMFrontSSC', 'ThreeActuatorAWD2EMRearSSC', 'TwoActuatorAWDSSC'}  VariantControlMode=label  VariantControl=Choice  LabelModeActiveChoice=OneActuatorFWDSSC
  Front Axle : Subsystem  Variant=on  VariantChoicesSpecifier={'DualEMDriveFrontSSC', 'LimitedSlipDifferentialSSC', 'NoDifferentialFrontSSC', 'OpenDifferentialSSC'}  VariantControlMode=label  VariantControl=Choice  LabelModeActiveChoice=OpenDifferentialSSC
  Rear Axle : Subsystem  Variant=on  VariantChoicesSpecifier={'DualEMDriveRear3EMSSC', 'DualEMDriveRear4EMSSC', 'LimitedSlipDifferentialSSC', 'NoDifferentialRearSSC', 'OpenDifferentialSSC'}  VariantControlMode=label  VariantControl=Choice  LabelModeActiveChoice=NoDifferentialRearSSC
      settings: PortSchema="{\"entries\":[{\"content\":{\"sides\":[{\"content\":{\"connectorIds\":[\"LConn1\",\"In1\",\"In2\"]},\"type\":\"ConnectorPlacement.EquallySpacedRectSide\",\"uuid\":\"74f8b1d8-6b3a-4eeb-b984-715de40eb708\"},{\"content\":{\"connectorIds\":[\"Out1\",\"Out2\",\"Out3\",\"Out4\",\"RConn1\",\"RConn2\"],\"side\":\"RIGHT\"},\"type\":\"ConnectorPlacement.EquallySpacedRectSide\",\"uuid\":\"c00021b1-b8b4-4ff3-9b35-429da9caaad3\"},{\"content\":{\"connectorIds\":[],\"side\":\"TOP\"},\"type\":\"ConnectorPlacement.EquallySpacedRectSide\",\"uuid\":\"0bf4e327-a693-4202-b285-43d08d42df4d\"}]},\"type\":\"ConnectorPlacement.EquallySpacedConnector\",\"uuid\":\"b41f4b2c-0e15-48ba-ac2c-145a8c4b8844\"}],\"packageUris\":[\"http://schema.mathworks.com/mf0/Connector/R2020b\"],\"version\":\"1.0\"}"
  Selector : Selector  InputPortWidth=4  IndexOptions=Index vector (dialog)  Indices=[3 4]  OutputSizes=1
  Selector1 : Selector  InputPortWidth=4  IndexOptions=Index vector (dialog)  Indices=[1 2]  OutputSizes=1
  Simscape Bus : SimscapeBus  HierarchyStrings=AxlFL;AxlFR;AxlRL;AxlRR
  Terminator{1..8} (8 alike) : Terminator
  DriveshftTrq : PMIOPort  Side=Left
  Axl : PMIOPort  Port=2  Side=Right
  DriveshftSpd : Outport  VectorParamsAs1DForOutWhenUnconnected=off
  AxlTrq : Outport  Port=2  VectorParamsAs1DForOutWhenUnconnected=off
  wires:
  Selector/1 -> Demux2/1
  Demux1/2 -> Front Axle/2(Prs2)
  Demux1/1 -> Front Axle/1(Prs1)
  Selector1/1 -> Demux1/1
  DiffrntlPrsCmd/1 -> Selector1/1, Selector/1
  Rear Axle/1(Info) -> Terminator5/1
  Front Axle/1(Info) -> Terminator1/1
  Demux2/1 -> Rear Axle/1(Prs1)
  Demux2/2 -> Rear Axle/2(Prs2)
  Front Axle/2(DriveshftSpd) -> Terminator2/1
  Front Axle/3(Axl1Spd) -> Terminator3/1
  Front Axle/4(Axl2Spd) -> Terminator4/1
  Rear Axle/2(DriveshftSpd) -> Terminator6/1
  Rear Axle/3(Axl1Spd) -> Terminator7/1
  Rear Axle/4(Axl2Spd) -> Terminator8/1
  Constant/1 -> Axle Interconnect/1(SplitRatio)
  Constant1/1 -> Axle Interconnect/2(Lockup)
  [T4] -> Bus Creator/4  "RR"
  [T3] -> Bus Creator/3  "RL"
  [T2] -> Bus Creator/2  "FR"
  [T1] -> Bus Creator/1  "FL"
  AxlTrqFL/1(Trq) -> [T1]
  AxlTrqFR/1(Trq) -> [T2]
  AxlTrqRL/1(Trq) -> [T3]
  AxlTrqR/1(Trq) -> [T4]
  DriveshftTrq Routing/1(DriveshftSpd) -> DriveshftSpd/1
  Bus Creator/1 -> AxlTrq/1
  connections:
  Simscape Bus/RConn1 -- Axl/RConn1
  Front Axle/RConn1 -- AxlTrqFL/LConn1
  Front Axle/RConn2 -- AxlTrqFR/LConn1
  Rear Axle/RConn2 -- AxlTrqR/LConn1
  Rear Axle/RConn1 -- AxlTrqRL/LConn1
  DriveshftTrq Routing/RConn1 -- Front Axle/LConn1
  DriveshftTrq Routing/RConn5 -- Rear Axle/LConn1
  Axle Interconnect/LConn1 -- DriveshftTrq Routing/RConn2
  Axle Interconnect/LConn2 -- DriveshftTrq Routing/RConn3
  Axle Interconnect/LConn3 -- DriveshftTrq Routing/RConn4
  AxlTrqFL/RConn1 -- Simscape Bus/LConn1
  AxlTrqFR/RConn1 -- Simscape Bus/LConn2
  AxlTrqRL/RConn1 -- Simscape Bus/LConn3
  AxlTrqR/RConn1 -- Simscape Bus/LConn4
  DriveshftTrq/RConn1 -- DriveshftTrq Routing/LConn1

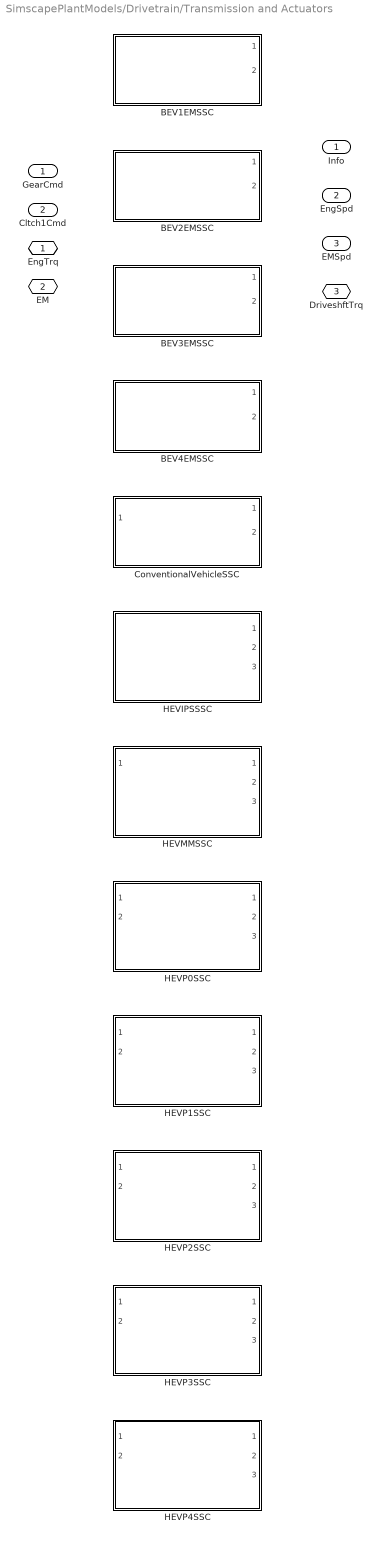
== system SimscapePlantModels/Drivetrain/Transmission and Actuators ==
  GearCmd : Inport
  Cltch1Cmd : Inport  Port=2
  BEV1EMSSC : Subsystem  VariantControl=BEV1EMSSC  ReferencedSubsystem=BEV1EMSSC
  BEV2EMSSC : Subsystem  VariantControl=BEV2EMSSC  ReferencedSubsystem=BEV2EMSSC
  BEV3EMSSC : Subsystem  VariantControl=BEV3EMSSC  ReferencedSubsystem=BEV3EMSSC
  BEV4EMSSC : Subsystem  VariantControl=BEV4EMSSC  ReferencedSubsystem=BEV4EMSSC
  ConventionalVehicleSSC : Subsystem  VariantControl=ConventionalVehicleSSC  ReferencedSubsystem=ConventionalVehicleSSC
  HEVIPSSSC : Subsystem  VariantControl=HEVIPSSSC  ReferencedSubsystem=HEVIPSSSC
  HEVMMSSC : Subsystem  VariantControl=HEVMMSSC  ReferencedSubsystem=HEVMMSSC
  HEVP0SSC : Subsystem  VariantControl=HEVP0SSC  ReferencedSubsystem=HEVP0SSC
  HEVP1SSC : Subsystem  VariantControl=HEVP1SSC  ReferencedSubsystem=HEVP1SSC
  HEVP2SSC : Subsystem  VariantControl=HEVP2SSC  ReferencedSubsystem=HEVP2SSC
  HEVP3SSC : Subsystem  VariantControl=HEVP3SSC  ReferencedSubsystem=HEVP3SSC
  HEVP4SSC : Subsystem  VariantControl=HEVP4SSC  ReferencedSubsystem=HEVP4SSC
  EngTrq : PMIOPort  Side=Left
  EM : PMIOPort  Port=2  Side=Left
  DriveshftTrq : PMIOPort  Port=3  Side=Right
  Info : Outport  VectorParamsAs1DForOutWhenUnconnected=off
  EngSpd : Outport  Port=2  VectorParamsAs1DForOutWhenUnconnected=off
  EMSpd : Outport  Port=3  VectorParamsAs1DForOutWhenUnconnected=off  BusOutputAsStruct=on

== system SimscapePlantModels/Pedal, Cluster, Cabin/Brake Pedal ==
  DecelCmd : Inport
  Dead Zone1 : DeadZone  LowerValue=0  UpperValue=.01  ZeroCross=off
  DecelFdbk : Outport
  wires:
  Dead Zone1/1 -> DecelFdbk/1
  DecelCmd/1 -> Dead Zone1/1

== system SimscapePlantModels/Sensors/Sensors ==
  VehFdbk : Inport
  IMUSensor : Subsystem  VariantControl=IMUSensor  ReferencedSubsystem=IMUSensor
  NoIMUSensor : Subsystem  VariantControl=NoIMUSensor  ReferencedSubsystem=NoIMUSensor
  IMU : Outport

== system SimscapePlantModels/Thermal/Electrical Cooling ==
  ValveCmd : Inport
  VehBody : Inport  Port=2
  AmbTmp : Inport  Port=3
  PumpCmd : Inport  Port=4
  Electrical Cooling System : Subsystem  VariantControl=Electrical Cooling System  ReferencedSubsystem=ElectricalCoolingSystemSSC
  No Thermal Effect : Subsystem  VariantControl=No Thermal Effect  ReferencedSubsystem=NoThermalEffectSSC
  ThrmElec : PMIOPort  Side=Left
  Thermal : Outport

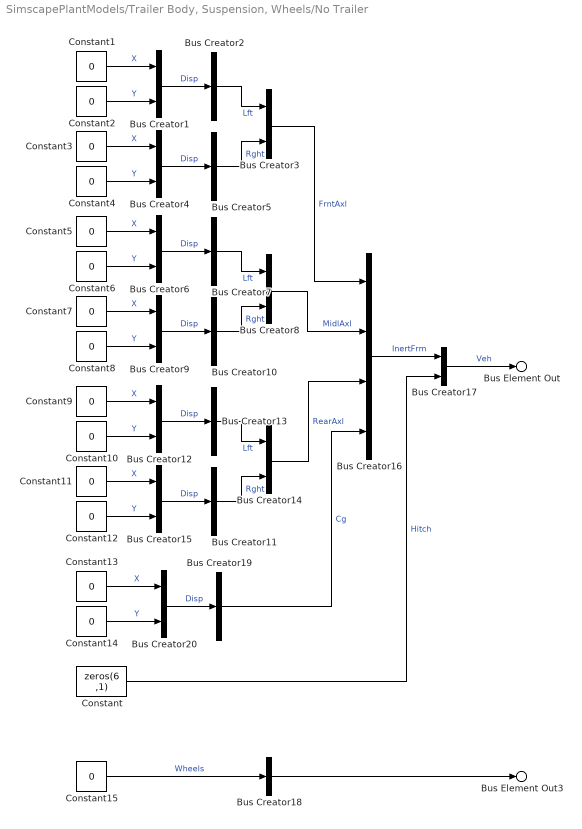
== system SimscapePlantModels/Trailer Body, Suspension, Wheels/No Trailer ==
  Bus Creator{1,3..4,6,8..9,12,14..15,17,20} (11 alike) : BusCreator  Inputs=2
  Bus Creator{2,5,7,10..11,13,18..19} (8 alike) : BusCreator  Inputs=1
  Bus Creator16 : BusCreator  Inputs=4
  Constant : Constant  Value=zeros(6 ,1)  SampleTime=-1
  Constant{1..15} (15 alike) : Constant  Value=0  SampleTime=-1
  Bus Element Out3 : Outport  PortName=Wheels
  Bus Element Out : Outport  Port=2  PortName=Veh
  wires:
  Constant1/1 -> Bus Creator1/1  "X"
  Bus Creator18/1 -> Bus Element Out3/1
  Constant2/1 -> Bus Creator1/2  "Y"
  Bus Creator1/1 -> Bus Creator2/1  "Disp"
  Bus Creator4/1 -> Bus Creator5/1  "Disp"
  Constant4/1 -> Bus Creator4/2  "Y"
  Constant3/1 -> Bus Creator4/1  "X"
  Bus Creator5/1 -> Bus Creator3/2  "Rght"
  Bus Creator2/1 -> Bus Creator3/1  "Lft"
  Bus Creator7/1 -> Bus Creator8/1  "Lft"
  Bus Creator10/1 -> Bus Creator8/2  "Rght"
  Constant7/1 -> Bus Creator9/1  "X"
  Constant8/1 -> Bus Creator9/2  "Y"
  Bus Creator9/1 -> Bus Creator10/1  "Disp"
  Bus Creator6/1 -> Bus Creator7/1  "Disp"
  Constant6/1 -> Bus Creator6/2  "Y"
  Constant5/1 -> Bus Creator6/1  "X"
  Constant9/1 -> Bus Creator12/1  "X"
  Constant10/1 -> Bus Creator12/2  "Y"
  Bus Creator12/1 -> Bus Creator13/1  "Disp"
  Bus Creator15/1 -> Bus Creator11/1  "Disp"
  Constant12/1 -> Bus Creator15/2  "Y"
  Constant11/1 -> Bus Creator15/1  "X"
  Bus Creator11/1 -> Bus Creator14/2  "Rght"
  Bus Creator13/1 -> Bus Creator14/1  "Lft"
  Bus Creator8/1 -> Bus Creator16/2  "MidlAxl"
  Bus Creator14/1 -> Bus Creator16/3  "RearAxl"
  Bus Creator3/1 -> Bus Creator16/1  "FrntAxl"
  Bus Creator16/1 -> Bus Creator17/1  "InertFrm"
  Bus Creator17/1 -> Bus Element Out/1  "Veh"
  Constant15/1 -> Bus Creator18/1  "Wheels"
  Bus Creator19/1 -> Bus Creator16/4  "Cg"
  Constant13/1 -> Bus Creator20/1  "X"
  Constant14/1 -> Bus Creator20/2  "Y"
  Bus Creator20/1 -> Bus Creator19/1  "Disp"
  Constant/1 -> Bus Creator17/2  "Hitch"

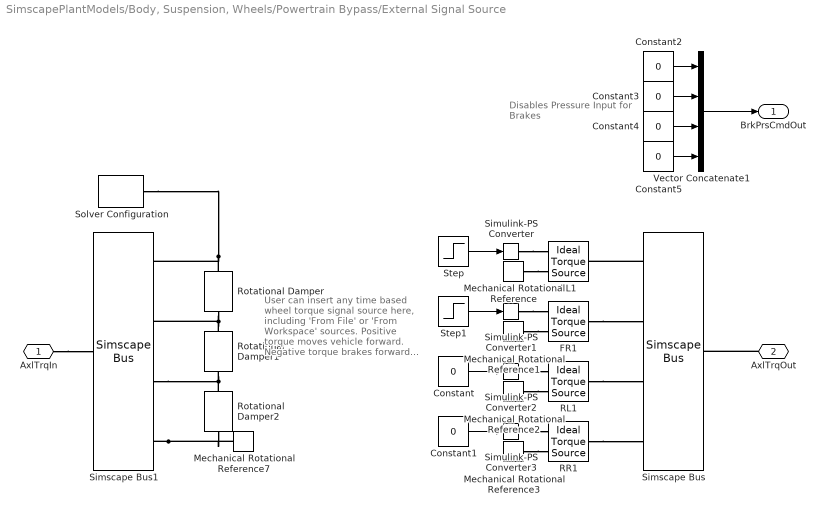
== system SimscapePlantModels/Body, Suspension, Wheels/Powertrain Bypass/External Signal Source ==
  note: User can insert any time based
      | wheel torque signal source here,
      | including 'From File' or 'From
      | Workspace' sources.
      |
      | Positive torque moves vehicle
      | forward.
      | Negative torque brakes forward
      | moving vehicle or moves vehicle
      | in reverse.
  note: Disables Pressure
      | Input for Brakes
  Constant{,1..5} (6 alike) : Constant  Value=0  SampleTime=-1
  FL1 : fl_lib/Mechanical/Mechanical Sources/Ideal Torque Source
  FR1 : fl_lib/Mechanical/Mechanical Sources/Ideal Torque Source
  Mechanical Rotational Reference{,1..3,7} (5 alike) : fl_lib/Mechanical/Rotational Elements/Mechanical Rotational Reference
  RL1 : fl_lib/Mechanical/Mechanical Sources/Ideal Torque Source
  RR1 : fl_lib/Mechanical/Mechanical Sources/Ideal Torque Source
  Rotational Damper : sdl_lib/Couplings & Drives/Springs & Dampers/Rotational Damper  D=1e5 N*m*s/rad  enable_faults=simscape.enum.onoff.off  b_fault=100 N*m*s/rad  temporal_fault=simscape.enum.onoff.off  fault_time=5 s  shock_fault=simscape.enum.onoff.off  acceleration_limit=100 rad/s^2  shock_limit=1  report_fault=simscape.enum.assert.action.none  thermal_port=simscape.enum.thermaleffects.omit  thermal_mass=50 kJ/K  temperature_specify=off  temperature_priority=High  temperature=300 K  temperature_nominal_specify=off  temperature_nominal_unit=K  temperature_nominal_value=1
  Rotational Damper1 : sdl_lib/Couplings & Drives/Springs & Dampers/Rotational Damper  D=1e5 N*m*s/rad  enable_faults=simscape.enum.onoff.off  b_fault=100 N*m*s/rad  temporal_fault=simscape.enum.onoff.off  fault_time=5 s  shock_fault=simscape.enum.onoff.off  acceleration_limit=100 rad/s^2  shock_limit=1  report_fault=simscape.enum.assert.action.none  thermal_port=simscape.enum.thermaleffects.omit  thermal_mass=50 kJ/K  temperature_specify=off  temperature_priority=High  temperature=300 K  temperature_nominal_specify=off  temperature_nominal_unit=K  temperature_nominal_value=1
  Rotational Damper2 : sdl_lib/Couplings & Drives/Springs & Dampers/Rotational Damper  D=1e5 N*m*s/rad  enable_faults=simscape.enum.onoff.off  b_fault=100 N*m*s/rad  temporal_fault=simscape.enum.onoff.off  fault_time=5 s  shock_fault=simscape.enum.onoff.off  acceleration_limit=100 rad/s^2  shock_limit=1  report_fault=simscape.enum.assert.action.none  thermal_port=simscape.enum.thermaleffects.omit  thermal_mass=50 kJ/K  temperature_specify=off  temperature_priority=High  temperature=300 K  temperature_nominal_specify=off  temperature_nominal_unit=K  temperature_nominal_value=1
  Simscape Bus : SimscapeBus  HierarchyStrings=AxlFL;AxlFR;AxlRL;AxlRR
  Simscape Bus1 : SimscapeBus  HierarchyStrings=AxlFL;AxlFR;AxlRL;AxlRR
  Simulink-PS Converter{,1..3} (4 alike) : nesl_utility_internal/Simulink-PS Converter  PhysicalDomain=network_engine_domain  SubClassName=ps_input  LeftPortType=input  RightPortType=output  PseudoPeriodic=off  Frequencies=[]  NoiseDistribution=none  NoiseParameters=[]  Unit=1  AffineConversion=off  FilteringAndDerivatives=provide  SimscapeFilterOrder=1  InputFilterTimeConstant=0.001  UdotUserProvided=0
  Solver Configuration : nesl_utility_internal/Solver Configuration  PhysicalDomain=network_engine_domain  SubClassName=solver  LeftPortType=input  RightPortType=generic  Tones=[]  Harmonics=[]  SimulateNoise=off  Profile=off  UseLocalSampling=off  EnableSwitchedLinearOptims=on  FrequencyDomain=off  UseCCode=off  RelTol=0.001  AbsTol=0.001  MinStep=1e-09  ToWorkspace=off  RevertToSquareIcSolve=off  NumHomotopyIterations=100  PhasorMode=off  PhasorModeNumHarmonics=1  ConsistencySolver=NEWTON_XTOL_AFTER_FTOL  IndexReductionMethod=DerivativeReplacement  DoDC=off  ResidualTolerance=1e-09  ConsistencyTolSource=GLOBAL  ConsistencyAbsTol=0.001  ConsistencyRelTol=0.001  ConsistencyTolFactor=0.001  UseLocalSolver=off  LocalSolverChoice=NE_BACKWARD_EULER_ADVANCER  ResolveIndetEquations=on  FunctionEvalNumThread=1  LocalSolverSampleTime=0.001  DoFixedCost=off  MaxNonlinIter=3  MaxModeIter=2  ComputeImpulses=off  ImpulseIterations=2  LinearAlgebra=auto  LinearAlgebraNumThread=0  EquationFormulation=NE_TIME_EF  DelaysMemoryBudget=1024  AutomaticFiltering=on  FilteringTimeConstant=0.001  PartitionStorageMethod=AS_NEEDED  PartitionMemoryBudget=1024  PartitionMethod=ROBUST  MultibodyUseLocalSolver=off  MultibodyLocalSolverChoice=ODE1  MultibodyLocalSolverSampleTime=0.001
  Step : Step  After=100  SampleTime=0
  Step1 : Step  After=100  SampleTime=0
  Vector Concatenate1 : Concatenate  NumInputs=4
  AxlTrqIn : PMIOPort  Side=Left
  AxlTrqOut : PMIOPort  Port=2  Side=Right
  BrkPrsCmdOut : Outport
  wires:
  Constant2/1 -> Vector Concatenate1/1
  Constant3/1 -> Vector Concatenate1/2
  Constant4/1 -> Vector Concatenate1/3
  Vector Concatenate1/1 -> BrkPrsCmdOut/1
  Constant5/1 -> Vector Concatenate1/4
  Step1/1 -> Simulink-PS Converter1/1
  Step/1 -> Simulink-PS Converter/1
  Constant1/1 -> Simulink-PS Converter3/1
  Constant/1 -> Simulink-PS Converter2/1
  connections:
  Rotational Damper/LConn1 -- Simscape Bus1/LConn1 -- Solver Configuration/RConn1
  Rotational Damper2/LConn1 -- Simscape Bus1/LConn3 -- Rotational Damper1/RConn1
  Simscape Bus1/LConn4 -- Rotational Damper2/RConn1 -- Mechanical Rotational Reference7/LConn1
  Rotational Damper1/LConn1 -- Rotational Damper/RConn1 -- Simscape Bus1/LConn2
  Simulink-PS Converter3/RConn1 -- RR1/RConn1
  AxlTrqOut/RConn1 -- Simscape Bus/RConn1
  RR1/LConn1 -- Simscape Bus/LConn4
  Mechanical Rotational Reference1/LConn1 -- FR1/RConn2
  FR1/LConn1 -- Simscape Bus/LConn2
  AxlTrqIn/RConn1 -- Simscape Bus1/RConn1
  Simulink-PS Converter2/RConn1 -- RL1/RConn1
  RL1/LConn1 -- Simscape Bus/LConn3
  Mechanical Rotational Reference/LConn1 -- FL1/RConn2
  Simulink-PS Converter/RConn1 -- FL1/RConn1
  Mechanical Rotational Reference3/LConn1 -- RR1/RConn2
  Simscape Bus/LConn1 -- FL1/LConn1
  Simulink-PS Converter1/RConn1 -- FR1/RConn1
  Mechanical Rotational Reference2/LConn1 -- RL1/RConn2

== system SimscapePlantModels/Body, Suspension, Wheels/Powertrain Bypass/Pass Through ==
  BrkPrsCmdIn : Inport
  AxlTrqIn : PMIOPort  Side=Left
  AxlTrqOut : PMIOPort  Port=2  Side=Right
  BrkPrsCmdOut : Outport
  wires:
  BrkPrsCmdIn/1 -> BrkPrsCmdOut/1
  connections:
  AxlTrqOut/RConn1 -- AxlTrqIn/RConn1

== system SimscapePlantModels/Drivetrain/Drivetrain Layout/AxlTrqFL ==
  Ideal Torque Sensor : fl_lib/Mechanical/Mechanical Sensors/Ideal Torque Sensor
  PS-Simulink Converter : nesl_utility_internal/PS-Simulink Converter  PhysicalDomain=network_engine_domain  SubClassName=ps_output  LeftPortType=input  RightPortType=output  PseudoPeriodic=off  Frequencies=[]  VectorFormat=inherit  Unit=inherit  AffineConversion=off
  R : PMIOPort  Side=Left
  C : PMIOPort  Port=2  Side=Right
  Trq : Outport
  wires:
  PS-Simulink Converter/1 -> Trq/1
  connections:
  Ideal Torque Sensor/LConn1 -- R/RConn1
  Ideal Torque Sensor/RConn1 -- C/RConn1
  PS-Simulink Converter/LConn1 -- Ideal Torque Sensor/RConn2

== system SimscapePlantModels/Drivetrain/Drivetrain Layout/AxlTrqFR ==
  Ideal Torque Sensor : fl_lib/Mechanical/Mechanical Sensors/Ideal Torque Sensor
  PS-Simulink Converter : nesl_utility_internal/PS-Simulink Converter  PhysicalDomain=network_engine_domain  SubClassName=ps_output  LeftPortType=input  RightPortType=output  PseudoPeriodic=off  Frequencies=[]  VectorFormat=inherit  Unit=inherit  AffineConversion=off
  R : PMIOPort  Side=Left
  C : PMIOPort  Port=2  Side=Right
  Trq : Outport
  wires:
  PS-Simulink Converter/1 -> Trq/1
  connections:
  PS-Simulink Converter/LConn1 -- Ideal Torque Sensor/RConn2
  Ideal Torque Sensor/RConn1 -- C/RConn1
  Ideal Torque Sensor/LConn1 -- R/RConn1

== system SimscapePlantModels/Drivetrain/Drivetrain Layout/AxlTrqR ==
  Ideal Torque Sensor : fl_lib/Mechanical/Mechanical Sensors/Ideal Torque Sensor
  PS-Simulink Converter : nesl_utility_internal/PS-Simulink Converter  PhysicalDomain=network_engine_domain  SubClassName=ps_output  LeftPortType=input  RightPortType=output  PseudoPeriodic=off  Frequencies=[]  VectorFormat=inherit  Unit=inherit  AffineConversion=off
  R : PMIOPort  Side=Left
  C : PMIOPort  Port=2  Side=Right
  Trq : Outport
  wires:
  PS-Simulink Converter/1 -> Trq/1
  connections:
  PS-Simulink Converter/LConn1 -- Ideal Torque Sensor/RConn2
  Ideal Torque Sensor/RConn1 -- C/RConn1
  Ideal Torque Sensor/LConn1 -- R/RConn1
